simulink model "motorthrust"  (R2017b)
settings: Solver=FixedStepAuto  StartTime=0.0  StopTime=10.0  FixedStep=interval  RelTol=1e-3
values from neighbouring files (symbols this model uses):
  b = 0.01    [Motor_Parameters.m]
  d = 20    [Motor_Parameters.m]    (also in Quad_vis.m = 1)
  J = 0.0007    [Motor_Parameters.m]
  Ke = 0.0734    [Motor_Parameters.m]
  Kt = 0.076    [Motor_Parameters.m]
  L = 0.000224    [Motor_Parameters.m]
  pitch = 7    [Motor_Parameters.m]
  R = 0.000230    (= 0.00023)    [Motor_Parameters.m]    (also in elevation_lin_script.m = 1; pitch_lin_script.m = 1; roll_lin_script.m = 1; yaw_lin_script.m = 1)
  V_bat = 44.4    [Motor_Parameters.m]
  x1 = 4.392399*10^-8    (= 4.392399e-08)    [Motor_Parameters.m]
  x2 = 4.23333*10^-4    (= 0.000423333)    [Motor_Parameters.m]
libraries: simulink x1
settings Model: Creator=DanAdmin  LastModifiedBy=schapman

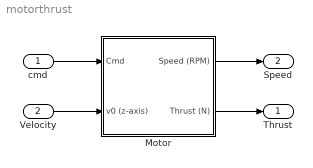
== system motorthrust ==
  cmd : Inport
  Velocity : Inport  Port=2
  Motor : Subsystem
  Thrust : Outport
  Speed : Outport  Port=2
  wires:
  cmd/1 -> Motor/1(Cmd)
  Motor/2(Thrust (N)) -> Thrust/1
  Motor/1(Speed (RPM)) -> Speed/1
  Velocity/1 -> Motor/2(v0 (z-axis))

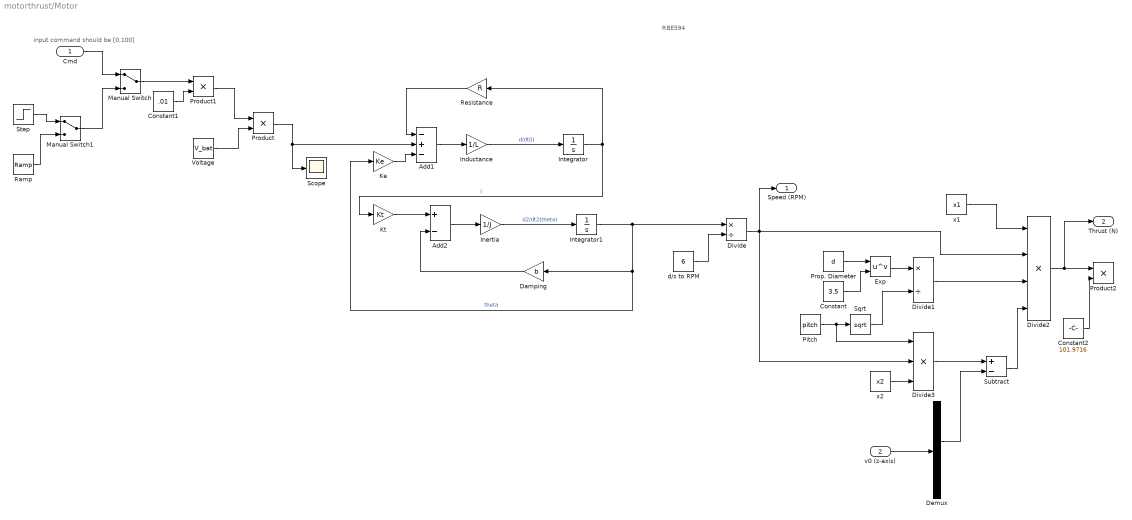
== system motorthrust/Motor ==
  note: input command should be [0,100]
  note: RBE594
  Cmd : Inport  OutMin=[0]  OutMax=[100]
  v0 (z-axis) : Inport  Port=2  OutMin=[0]  OutMax=[1]
  Add1 : Sum  Inputs=-+-
  Add2 : Sum  Inputs=+-
  Constant : Constant  Value=3.5
  Constant1 : Constant  Value=.01
  Constant2 : Constant  Value=101.9716
  Damping : Gain  Gain=b
  Demux : Demux  Outputs=6
  Divide : Product  Inputs=*/
  Divide1 : Product  Inputs=*/
  Divide2 : Product  Inputs=****
  Divide3 : Product  Inputs=***
  Exp : Math  Operator=pow  SaturateOnIntegerOverflow=on
  Inductance : Gain  Gain=1/L
  Inertia : Gain  Gain=1/J
  Integrator : Integrator
  Integrator1 : Integrator
  Ke : Gain  Gain=Ke
  Kt : Gain  Gain=Kt
  Manual Switch : ManualSwitch
  Manual Switch1 : ManualSwitch
  Pitch : Constant  Value=pitch
  Product : Product
  Product1 : Product
  Product2 : Product
  Prop. Diameter : Constant  Value=d
  Ramp : simulink/Sources/Ramp  slope=15  start=1  X0=0
  Resistance : Gain  Gain=R
  Scope : Scope
  Sqrt : Sqrt  SaturateOnIntegerOverflow=on
  Step : Step  After=100  SampleTime=0
  Subtract : Sum  Inputs=+-
  Voltage : Constant  Value=V_bat
  d/s to RPM : Constant  Value=6
  x1 : Constant  Value=x1
  x2 : Constant  Value=x2
  Speed (RPM) : Outport
  Thrust (N) : Outport  Port=2
  wires:
  Inductance/1 -> Integrator/1  "d/dt(i)"
  Integrator/1 -> Resistance/1, Kt/1  "i"
  Integrator1/1 -> Divide/1, Ke/1, Damping/1  "theta"
  Inertia/1 -> Integrator1/1  "d2/dt2(theta)"
  Add1/1 -> Inductance/1
  Add2/1 -> Inertia/1
  Damping/1 -> Add2/2
  Kt/1 -> Add2/1
  Ke/1 -> Add1/3
  Resistance/1 -> Add1/1
  d/s to RPM/1 -> Divide/2
  Product/1 -> Scope/1, Add1/2
  Pitch/1 -> Divide3/1, Sqrt/1
  Subtract/1 -> Divide2/4
  Divide3/1 -> Subtract/1
  Sqrt/1 -> Divide1/2
  Constant/1 -> Exp/2
  Exp/1 -> Divide1/1
  x2/1 -> Divide3/3
  Divide1/1 -> Divide2/3
  Prop. Diameter/1 -> Exp/1
  x1/1 -> Divide2/1
  Divide/1 -> Divide3/2, Divide2/2, Speed (RPM)/1
  Voltage/1 -> Product/2
  Divide2/1 -> Thrust (N)/1, Product2/1
  Constant2/1 -> Product2/2
  Constant1/1 -> Product1/2
  Product1/1 -> Product/1
  v0 (z-axis)/1 -> Demux/1
  Demux/3 -> Subtract/2
  Manual Switch/1 -> Product1/1
  Cmd/1 -> Manual Switch/1
  Step/1 -> Manual Switch1/1
  Ramp/1 -> Manual Switch1/2
  Manual Switch1/1 -> Manual Switch/2
